simulink model "modele_mpc"  (R2026a)
settings: Solver=VariableStepAuto
values from neighbouring files (symbols this model uses):
  A_obs = A - L*C    [init_lqr.m]
  B_obs = [B, L]    [init_lqr.m]
  C_obs = eye(4)    [init_lqr.m]
  D_obs = zeros(4,3)    [init_lqr.m]
  GtQbarF = G' * Q_bar * F    [init_mpc.m]
  H_qp = (H_qp + H_qp') / 2    [init_mpc.m]    (also in mpc_blk.m = evalin('base', 'H_qp'))
  lb = u_min * ones(N, 1)    [init_mpc.m]    (also in mpc_blk.m = evalin('base', 'lb'))
  theta0 = pi*theta0/180    (= 0.174532925199)    [init_params.m]
  ub = u_max * ones(N, 1)    [init_mpc.m]    (also in mpc_blk.m = evalin('base', 'ub'))
settings Model: Creator=floberg  LastModifiedBy=floberg

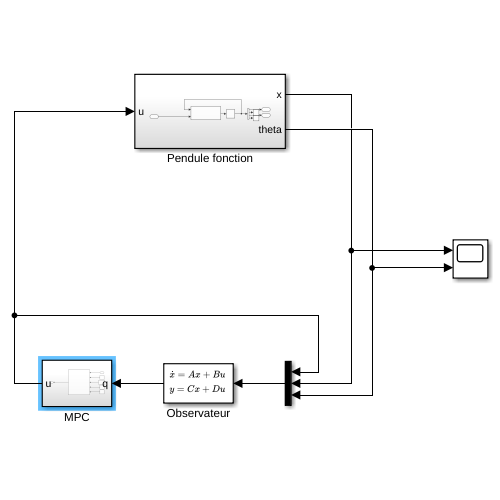
[thumbnail: Simulink's stored preview of the top-level diagram]
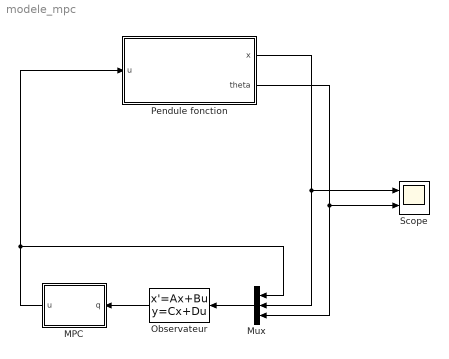
== system modele_mpc ==
  MPC : Subsystem
  Mux : Mux  Inputs=3
  Observateur : StateSpace  A=A_obs  B=B_obs  C=C_obs  D=D_obs  InitialCondition=0
  Pendule fonction : Subsystem
  Scope : Scope  NumInputPorts=2
      settings: ActiveDisplayYMinimum=-1.7225360374625065  ActiveDisplayYMaximum=1.0797563234132292
  wires:
  Mux/1 -> Observateur/1
  Pendule fonction/2(theta) -> Mux/3, Scope/2
  Pendule fonction/1(x) -> Scope/1, Mux/2
  MPC/1(u) -> Mux/1, Pendule fonction/1(u)
  Observateur/1 -> MPC/1(q)

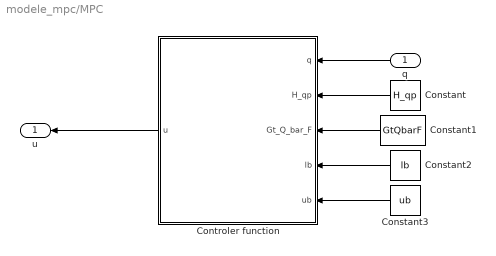
== system modele_mpc/MPC ==
  q : Inport
  Constant : Constant  Value=H_qp
  Constant1 : Constant  Value=GtQbarF
  Constant2 : Constant  Value=lb
  Constant3 : Constant  Value=ub
  Controler function : MATLAB Function  TreatAsAtomicUnit=on
  u : Outport
  wires:
  Constant2/1 -> Controler function/4(lb)
  Constant3/1 -> Controler function/5(ub)
  Constant/1 -> Controler function/2(H_qp)
  Constant1/1 -> Controler function/3(Gt_Q_bar_F)
  Controler function/1(u) -> u/1
  q/1 -> Controler function/1(q)

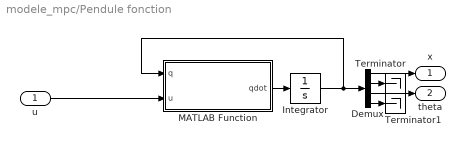
== system modele_mpc/Pendule fonction ==
  u : Inport
  Demux : Demux
  Integrator : Integrator  InitialCondition=[0;0;theta0;0]  UpperSaturationLimit=[100;100;6;100]  LowerSaturationLimit=[-100;-100;-6;-100]
  MATLAB Function : MATLAB Function  TreatAsAtomicUnit=on
  Terminator : Terminator
  Terminator1 : Terminator
  x : Outport
  theta : Outport  Port=2
  wires:
  Integrator/1 -> MATLAB Function/1(q), Demux/1
  Demux/3 -> theta/1
  MATLAB Function/1(qdot) -> Integrator/1
  Demux/1 -> x/1
  u/1 -> MATLAB Function/2(u)
  Demux/2 -> Terminator/1
  Demux/4 -> Terminator1/1

== matlab function modele_mpc/MPC/Controler function ==
  data: q input; u output; H_qp input; Gt_Q_bar_F input; lb input; ub input
function u = MPC_block(q, H_qp, Gt_Q_bar_F, lb, ub)
    % H_qp    : (N x N)     — hessien pré-calculé
    % Q_bar_F : (N*nx x nx) — produit G'*Q_bar*F pré-calculé
    % lb, ub  : (N x 1)     — bornes sur U

    % Déclarer quadprog comme extrinsèque (pas de codegen)
    coder.extrinsic('quadprog');
    
    % Initialisation de u
    N   = numel(lb);
    U_opt = zeros(N, 1); % Initialisé à zero pour

    % Gradient (dépend de q courant)
    f_qp = Gt_Q_bar_F * q;    

    % Résolution QP — initialiser U_opt obligatoire pour codegen
    U_opt = zeros(size(lb));
    U_opt = quadprog(H_qp, f_qp, [], [], [], [], lb, ub, U_opt, ...
                 optimoptions('quadprog', 'Display', 'off', ...
                              'Algorithm', 'active-set'));

    % Premier élément uniquement
    if isempty(U_opt)
        u = 0.0;
    else
        u = U_opt(1);
    end
end

== matlab function modele_mpc/Pendule fonction/MATLAB Function ==
  data: q input; u input; qdot output
function qdot = pendule_nonlineaire(q, u)
    % Paramètres
    M = 1.0; m = 0.1; l = 0.5; g = 9.81;

    x     = q(1);
    xdot  = q(2);
    theta = q(3);
    tdot  = q(4);  % theta_dot

    D = M + m*sin(theta)^2; % Dénominateur commun

    % Equations exactes non linéaires
    xddot = ( u + m*sin(theta)*(l*tdot^2 - g*cos(theta)) ) / D;

    tddot = ( -u*cos(theta) ...
              - m*l*tdot^2*sin(theta)*cos(theta) ...
              + (M+m)*g*sin(theta) ) / (l * D);

    qdot = [xdot; xddot; tdot; tddot];
end
